simulink model "FD_PITCH"  (R2019b)
settings: Solver=VariableStepAuto  StartTime=0.0  StopTime=10.0  RelTol=1e-3
undefined symbols (not defined in the file): Dm, Dt, g, Jp, k_pitch, Mb
libraries: cstblocks x2
settings Model: Creator=lbend  LastModifiedBy=peter

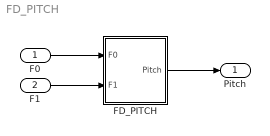
== system FD_PITCH ==
  F0 : Inport
  F1 : Inport  Port=2
  FD_PITCH : Subsystem
  Pitch : Outport
  wires:
  F0/1 -> FD_PITCH/1(F0)
  F1/1 -> FD_PITCH/2(F1)
  FD_PITCH/1(Pitch) -> Pitch/1

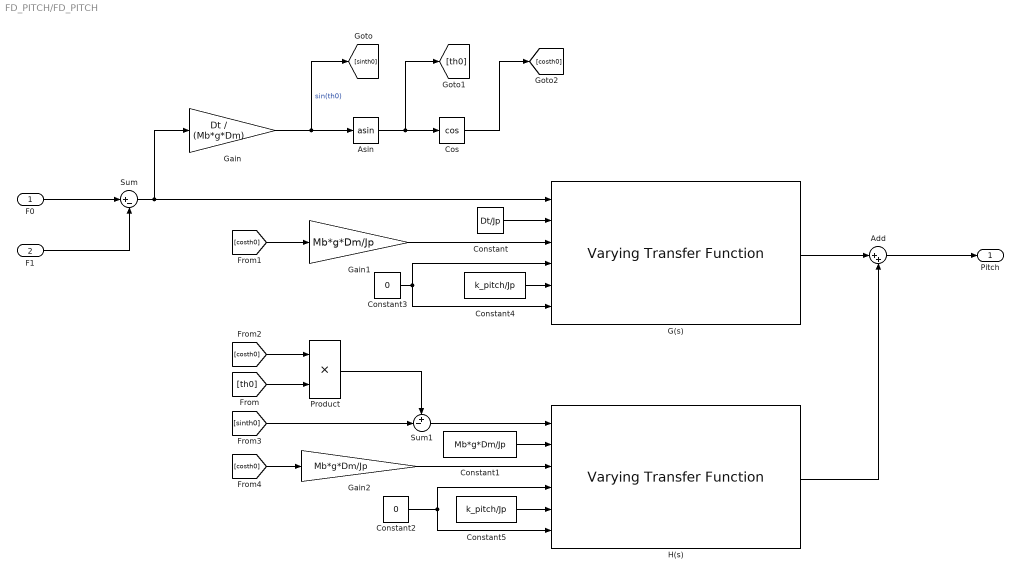
== system FD_PITCH/FD_PITCH ==
  F0 : Inport
  F1 : Inport  Port=2
  Add : Sum  Inputs=|++
  Asin : Trigonometry  Operator=asin
  Constant : Constant  Value=Dt/Jp
  Constant1 : Constant  Value=Mb*g*Dm/Jp
  Constant2 : Constant  Value=0
  Constant3 : Constant  Value=0
  Constant4 : Constant  Value=k_pitch/Jp
  Constant5 : Constant  Value=k_pitch/Jp
  Cos : Trigonometry  Operator=cos
  G(s) : cstblocks/Linear Parameter Varying/Varying Transfer Function  N=2
      settings: SourceProductName=Control System Toolbox
  Gain : Gain  Gain=Dt / (Mb*g*Dm)
  Gain1 : Gain  Gain=Mb*g*Dm/Jp
  Gain2 : Gain  Gain=Mb*g*Dm/Jp
  H(s) : cstblocks/Linear Parameter Varying/Varying Transfer Function  N=2
      settings: SourceProductName=Control System Toolbox
  Product : Product
  Sum : Sum  Inputs=|+-
  Sum1 : Sum  Inputs=+-|
  Pitch : Outport
  wires:
  F1/1 -> Sum/2
  Constant1/1 -> H(s)/2
  Gain/1 -> [sinth0], Asin/1  "sin(th0)"
  Constant2/1 -> H(s)/6, H(s)/4
  Asin/1 -> [th0], Cos/1
  Gain2/1 -> H(s)/3
  [sinth0] -> Sum1/2
  Sum/1 -> G(s)/1, Gain/1
  Constant4/1 -> G(s)/5
  Product/1 -> Sum1/1
  [costh0] -> Gain1/1
  [th0] -> Product/2
  H(s)/1 -> Add/2
  F0/1 -> Sum/1
  [costh0] -> Product/1
  Constant/1 -> G(s)/2
  Constant3/1 -> G(s)/6, G(s)/4
  Gain1/1 -> G(s)/3
  [costh0] -> Gain2/1
  Constant5/1 -> H(s)/5
  Cos/1 -> [costh0]
  G(s)/1 -> Add/1
  Sum1/1 -> H(s)/1
  Add/1 -> Pitch/1
